simulink model "trab1_questao3_linear"  (R2020a)
settings: Solver=VariableStepAuto  StartTime=0.0  StopTime=10.0  RelTol=1e-3
settings Model: Creator=luang  LastModifiedBy=luang

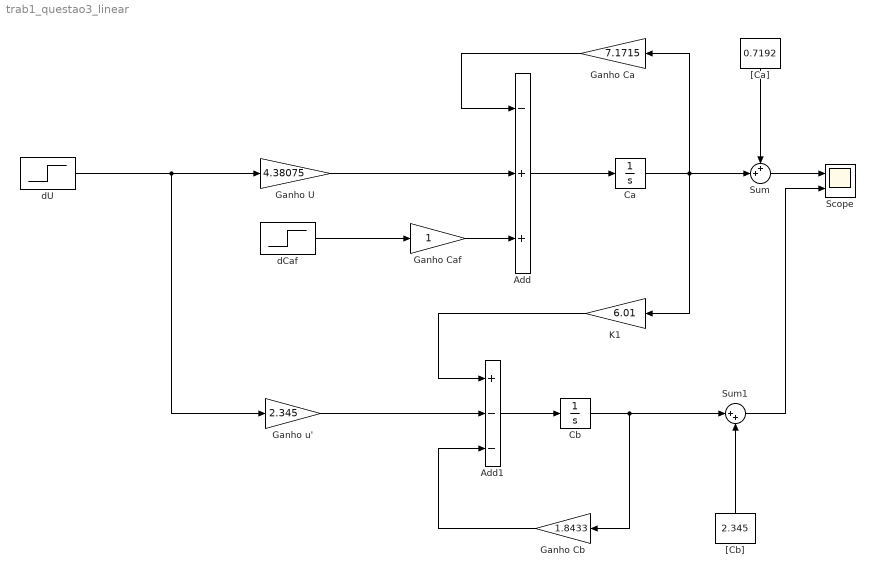
== system trab1_questao3_linear ==
  Add : Sum  Inputs=-++
  Add1 : Sum  Inputs=+--
  Ca : Integrator
  Cb : Integrator
  Ganho Ca : Gain  Gain=7.1715
  Ganho Caf : Gain
  Ganho Cb : Gain  Gain=1.8433
  Ganho U : Gain  Gain=4.38075
  Ganho u' : Gain  Gain=2.345
  K1 : Gain  Gain=6.01
  Scope : Scope  NumInputPorts=2
  Sum : Sum  Inputs=++|
  Sum1 : Sum  Inputs=|++
  "[Ca]" : Constant  Value=0.7192
  "[Cb]" : Constant  Value=2.345
  dCaf : Step  Time=0  After=0.1  SampleTime=0
  dU : Step  Time=0  After=0.1  SampleTime=0
  wires:
  Ganho u'/1 -> Add1/2
  Add/1 -> Ca/1
  Ganho Ca/1 -> Add/1
  dCaf/1 -> Ganho Caf/1
  Ganho Caf/1 -> Add/3
  Ca/1 -> Ganho Ca/1, K1/1, Sum/2
  Sum/1 -> Scope/1
  K1/1 -> Add1/1
  Ganho Cb/1 -> Add1/3
  Add1/1 -> Cb/1
  Cb/1 -> Ganho Cb/1, Sum1/1
  "[Cb]"/1 -> Sum1/2
  "[Ca]"/1 -> Sum/1
  dU/1 -> Ganho u'/1, Ganho U/1
  Ganho U/1 -> Add/2
  Sum1/1 -> Scope/2
